simulink model "DLCReferenceApplication"  (R2018a)
settings: Solver=ode23tb  StartTime=0.0  StopTime=20  FixedStep=.001  RelTol=5e-3  EnableMultiTasking=on
StartFcn:
  | %tic
StopFcn:
  | %toc
model workspace (MAT data in the model file):
  A_mu = 10
  B_reff = 8.386
  Cz = 7766.25
  DCT_Param : struct (value not decoded)
  D_reff = 0.25826
  Downshift_Speeds = [9.5625 12.9375 16.3125 19.6875 23.0625 26.4375 29.8125 33.1875 36.5625 39.9375 43.3125 46.6875 ... (28 elements, 4x7)]
  Pedal_Positions = [0.1 0.4 0.5 0.9]
  SUS : struct (value not decoded)
  Upshift_Speeds = [12.9375 16.3125 19.6875 33 26.4375 29.8125 33.1875 52.5 39.9375 43.3125 46.6875 77.25 ... (28 elements, 4x7)]
  VEH : struct (value not decoded)
  V_o = 16.7
  V_xlow = 1
  WH : struct (value not decoded)
  a = 1.4
  alpha_max = 1.5
  alpha_min = -1.5
  b = 1.8
  c_zo = 209651
  epsilon = 0.1
  h = 0.134
  path : struct (value not decoded)
  pio = 220000
  q_Fcx = 0
  q_Fz2 = 15.4
  q_Fzy = 0
  q_reo = 0.9974
  q_sx1 = -0.007764
  q_sx10 = 0.2824
  q_sx11 = 5.349
  q_sx12 = 0
  q_sx13 = 0
  q_sx14 = 0
  q_sx2 = 1.1915
  q_sx3 = 0.013948
  q_sx4 = 4.912
  q_sx5 = 1.02
  q_sx6 = 22.83
  q_sx7 = 0.7104
  q_sx8 = -0.023393
  q_sx9 = 0.6581
  q_sy1 = 0.00702
  q_sy2 = 0
  q_sy3 = 0.001515
  q_sy4 = 8.514e-05
  q_sy5 = 0
  q_sy6 = 0
  q_sy7 = 0.9008
  q_sy8 = -0.4089
  q_v1 = 0.0007742
  q_v2 = 0.04667
  r_Bx1 = 12.531
  r_Bx2 = 9.532
  r_Bx3 = 0
  r_By1 = 10.615
  r_By2 = 7.705
  r_By3 = 3.433e-06
  r_By4 = 0
  r_Cx1 = 1.019
  r_Cy1 = 1.0585
  r_Ex1 = -0.4487
  r_Ex2 = -0.4726
  r_Ey1 = 0.3132
  r_Ey2 = 7.63e-06
  r_Hx1 = 0.0002374
  r_Hy1 = 0.011646
  r_Hy2 = 7.63e-06
  r_Vy1 = 0.05654
  r_Vy2 = 7.63e-06
  r_Vy3 = 0
  r_Vy4 = 99.9
  r_Vy5 = 2
  r_Vy6 = 15.814
  r_o = 0.3135
  vehWidth = 2
  w = 1
symbols that are objects in the model workspace (value not decoded): VEH
libraries: neural x286, simulink x5, sim3dlib x2, autolibutils x1, vehdynlibscenariocommon x1, vehdynlibdriver x1, vehdynlibviscommon x1
(part 13 of 13)

== system DLCReferenceApplication/Predictive Driver/Model Prediction Net/Layer 4/Delays 1 ==
  "p{4}" : Inport  PortDimensions=9
      mask Display: e = 0.06;c1 = [120 230 180]/255;c2 = ([120 230 180]+0)/(256+128);c3 = ([120 230 180]+128)/(256+128);patch([0 1 1 0],[0 0 1 1],c1);patch([0 1 1 1-e 1-e 0+e],[0 0 1 1-e 0+e 0+e],c2);patch([0 0 1 1-e 0+e 0+e],[0 1 1 1-e 1-e 0+e],c3);plot([0 1 1 0 0],[0 0 1 1 0]);
  mux : Mux  Inputs=1
      mask Display: e = 0.06;c1 = [120 150 230]/255;c2 = ([120 150 230]+0)/383;c3 = ([120 150 230]+128)/383;patch([0 1 1 0],[0 0 1 1],c1);patch([0 1 1 1-e 1-e 0+e],[0 0 1 1-e 0+e 0+e],c2);patch([0 0 1 1-e 0+e 0+e],[0 1 1 1-e 1-e 0+e],c3);plot([0 1 1 0 0],[0 0 1 1 0]);disp('Mux')
  "pd{4,1}" : Outport
      mask Display: e = 0.06;c1 = [120 230 180]/255;c2 = ([120 230 180]+0)/(256+128);c3 = ([120 230 180]+128)/(256+128);patch([0 1 1 0],[0 0 1 1],c1);patch([0 1 1 1-e 1-e 0+e],[0 0 1 1-e 0+e 0+e],c2);patch([0 0 1 1-e 0+e 0+e],[0 1 1 1-e 1-e 0+e],c3);plot([0 1 1 0 0],[0 0 1 1 0]);
  wires:
  "p{4}"/1 -> mux/1
  mux/1 -> "pd{4,1}"/1

== system DLCReferenceApplication/Predictive Driver/Model Prediction Net/Layer 4/Delays 2 ==
  "p{4}" : Inport  PortDimensions=20
      mask Display: e = 0.06;c1 = [120 230 180]/255;c2 = ([120 230 180]+0)/(256+128);c3 = ([120 230 180]+128)/(256+128);patch([0 1 1 0],[0 0 1 1],c1);patch([0 1 1 1-e 1-e 0+e],[0 0 1 1-e 0+e 0+e],c2);patch([0 0 1 1-e 0+e 0+e],[0 1 1 1-e 1-e 0+e],c3);plot([0 1 1 0 0],[0 0 1 1 0]);
  mux : Mux  Inputs=1
      mask Display: e = 0.06;c1 = [120 150 230]/255;c2 = ([120 150 230]+0)/383;c3 = ([120 150 230]+128)/383;patch([0 1 1 0],[0 0 1 1],c1);patch([0 1 1 1-e 1-e 0+e],[0 0 1 1-e 0+e 0+e],c2);patch([0 0 1 1-e 0+e 0+e],[0 1 1 1-e 1-e 0+e],c3);plot([0 1 1 0 0],[0 0 1 1 0]);disp('Mux')
  "pd{4,1}" : Outport
      mask Display: e = 0.06;c1 = [120 230 180]/255;c2 = ([120 230 180]+0)/(256+128);c3 = ([120 230 180]+128)/(256+128);patch([0 1 1 0],[0 0 1 1],c1);patch([0 1 1 1-e 1-e 0+e],[0 0 1 1-e 0+e 0+e],c2);patch([0 0 1 1-e 0+e 0+e],[0 1 1 1-e 1-e 0+e],c3);plot([0 1 1 0 0],[0 0 1 1 0]);
  wires:
  "p{4}"/1 -> mux/1
  mux/1 -> "pd{4,1}"/1

== system DLCReferenceApplication/Predictive Driver/Model Prediction Net/Layer 4/Delays 3 ==
  "p{4}" : Inport  PortDimensions=40
      mask Display: e = 0.06;c1 = [120 230 180]/255;c2 = ([120 230 180]+0)/(256+128);c3 = ([120 230 180]+128)/(256+128);patch([0 1 1 0],[0 0 1 1],c1);patch([0 1 1 1-e 1-e 0+e],[0 0 1 1-e 0+e 0+e],c2);patch([0 0 1 1-e 0+e 0+e],[0 1 1 1-e 1-e 0+e],c3);plot([0 1 1 0 0],[0 0 1 1 0]);
  mux : Mux  Inputs=1
      mask Display: e = 0.06;c1 = [120 150 230]/255;c2 = ([120 150 230]+0)/383;c3 = ([120 150 230]+128)/383;patch([0 1 1 0],[0 0 1 1],c1);patch([0 1 1 1-e 1-e 0+e],[0 0 1 1-e 0+e 0+e],c2);patch([0 0 1 1-e 0+e 0+e],[0 1 1 1-e 1-e 0+e],c3);plot([0 1 1 0 0],[0 0 1 1 0]);disp('Mux')
  "pd{4,2}" : Outport
      mask Display: e = 0.06;c1 = [120 230 180]/255;c2 = ([120 230 180]+0)/(256+128);c3 = ([120 230 180]+128)/(256+128);patch([0 1 1 0],[0 0 1 1],c1);patch([0 1 1 1-e 1-e 0+e],[0 0 1 1-e 0+e 0+e],c2);patch([0 0 1 1-e 0+e 0+e],[0 1 1 1-e 1-e 0+e],c3);plot([0 1 1 0 0],[0 0 1 1 0]);
  wires:
  "p{4}"/1 -> mux/1
  mux/1 -> "pd{4,2}"/1

== system DLCReferenceApplication/Predictive Driver/Model Prediction Net/Layer 4/Delays 4 ==
  "p{4}" : Inport  PortDimensions=20
      mask Display: e = 0.06;c1 = [120 230 180]/255;c2 = ([120 230 180]+0)/(256+128);c3 = ([120 230 180]+128)/(256+128);patch([0 1 1 0],[0 0 1 1],c1);patch([0 1 1 1-e 1-e 0+e],[0 0 1 1-e 0+e 0+e],c2);patch([0 0 1 1-e 0+e 0+e],[0 1 1 1-e 1-e 0+e],c3);plot([0 1 1 0 0],[0 0 1 1 0]);
  mux : Mux  Inputs=1
      mask Display: e = 0.06;c1 = [120 150 230]/255;c2 = ([120 150 230]+0)/383;c3 = ([120 150 230]+128)/383;patch([0 1 1 0],[0 0 1 1],c1);patch([0 1 1 1-e 1-e 0+e],[0 0 1 1-e 0+e 0+e],c2);patch([0 0 1 1-e 0+e 0+e],[0 1 1 1-e 1-e 0+e],c3);plot([0 1 1 0 0],[0 0 1 1 0]);disp('Mux')
  "pd{4,3}" : Outport
      mask Display: e = 0.06;c1 = [120 230 180]/255;c2 = ([120 230 180]+0)/(256+128);c3 = ([120 230 180]+128)/(256+128);patch([0 1 1 0],[0 0 1 1],c1);patch([0 1 1 1-e 1-e 0+e],[0 0 1 1-e 0+e 0+e],c2);patch([0 0 1 1-e 0+e 0+e],[0 1 1 1-e 1-e 0+e],c3);plot([0 1 1 0 0],[0 0 1 1 0]);
  wires:
  "p{4}"/1 -> mux/1
  mux/1 -> "pd{4,3}"/1

== system DLCReferenceApplication/Predictive Driver/Model Prediction Net/Layer 4/IW{4,1} ==
  "pd{4,1}" : Inport  PortDimensions=9
      mask Display: e = 0.06;c1 = [120 230 180]/255;c2 = ([120 230 180]+0)/(256+128);c3 = ([120 230 180]+128)/(256+128);patch([0 1 1 0],[0 0 1 1],c1);patch([0 1 1 1-e 1-e 0+e],[0 0 1 1-e 0+e 0+e],c2);patch([0 0 1 1-e 0+e 0+e],[0 1 1 1-e 1-e 0+e],c3);plot([0 1 1 0 0],[0 0 1 1 0]);
  "IW{4,1}(1,:)'" : Constant  Value=[-0.5771230834189629010921862573013640940189361572265625;-0.61619201660164957257137530177715234458446502685546875;-0.3922129123495980973501673361170105636119842529296875;0.475137795096655823900988480090745724737644195556640625;0.207635780743493703059954214040772058069705963134765625;-0.391896217881100461521981515033985488116741180419921875;0.9160420222304281878678011707961559295654296875;0.2452005034204982891754553975260932929813861846923828125;-0.4981323816541636251287172854063101112842559814453125]
      mask Display: e = 0.06;c1 = [120 150 230]/255;c2 = ([120 150 230]+0)/383;c3 = ([120 150 230]+128)/383;patch([0 1 1 0],[0 0 1 1],c1);patch([0 1 1 1-e 1-e 0+e],[0 0 1 1-e 0+e 0+e],c2);patch([0 0 1 1-e 0+e 0+e],[0 1 1 1-e 1-e 0+e],c3);plot([0 1 1 0 0],[0 0 1 1 0]);disp('Weights');
  Mux : Mux  Inputs=1
      mask Display: e = 0.06;c1 = [120 150 230]/255;c2 = ([120 150 230]+0)/383;c3 = ([120 150 230]+128)/383;patch([0 1 1 0],[0 0 1 1],c1);patch([0 1 1 1-e 1-e 0+e],[0 0 1 1-e 0+e 0+e],c2);patch([0 0 1 1-e 0+e 0+e],[0 1 1 1-e 1-e 0+e],c3);plot([0 1 1 0 0],[0 0 1 1 0]);disp('Mux');
  dotprod1 : neural/Weight Functions/dotprod
  "iz{4,1}" : Outport
      mask Display: e = 0.06;c1 = [120 230 180]/255;c2 = ([120 230 180]+0)/(256+128);c3 = ([120 230 180]+128)/(256+128);patch([0 1 1 0],[0 0 1 1],c1);patch([0 1 1 1-e 1-e 0+e],[0 0 1 1-e 0+e 0+e],c2);patch([0 0 1 1-e 0+e 0+e],[0 1 1 1-e 1-e 0+e],c3);plot([0 1 1 0 0],[0 0 1 1 0]);
  wires:
  "IW{4,1}(1,:)'"/1 -> dotprod1/1
  "pd{4,1}"/1 -> dotprod1/2
  dotprod1/1 -> Mux/1
  Mux/1 -> "iz{4,1}"/1

== system DLCReferenceApplication/Predictive Driver/Model Prediction Net/Layer 4/LW{4,1} ==
  "ad{4,1}" : Inport  PortDimensions=20
      mask Display: e = 0.06;c1 = [120 230 180]/255;c2 = ([120 230 180]+0)/(256+128);c3 = ([120 230 180]+128)/(256+128);patch([0 1 1 0],[0 0 1 1],c1);patch([0 1 1 1-e 1-e 0+e],[0 0 1 1-e 0+e 0+e],c2);patch([0 0 1 1-e 0+e 0+e],[0 1 1 1-e 1-e 0+e],c3);plot([0 1 1 0 0],[0 0 1 1 0]);
  "IW{4,1}(1,:)'" : Constant  Value=[0.916684685790865483312472861143760383129119873046875;0.2636851771929895615897976313135586678981781005859375;-0.3492331089734814764113934870692901313304901123046875;-0.11786503709245825521900741250647115521132946014404296875;0.50320078446947380523823767362046055495738983154296875;-0.4927000401571077770057627276401035487651824951171875;-0.2088832457984179657994872059134650044143199920654296875;0.4465785632290864004545483112451620399951934814453125;0.10461125196919902891057319038736750371754169464111328125;-0.0427743850947984449728522804434760473668575286865234375;0.405797206791189746244441494127386249601840972900390625;-0.43662126395722722360659417972783558070659637451171875;-0.181658127076019193513189975419663824141025543212890625;0.41899883394469272790416880525299347937107086181640625;-0.533044452130733592554179267608560621738433837890625;0.16098318242033993197281915854546241462230682373046875;-0.219792476259432822960349085406051017343997955322265625;-0.426441538733121794368940982167259790003299713134765625;0.09693073801308534076515144306540605612099170684814453125;-0.0290423415959079438131151817970021511428058147430419921875]
      mask Display: e = 0.06;c1 = [120 150 230]/255;c2 = ([120 150 230]+0)/383;c3 = ([120 150 230]+128)/383;patch([0 1 1 0],[0 0 1 1],c1);patch([0 1 1 1-e 1-e 0+e],[0 0 1 1-e 0+e 0+e],c2);patch([0 0 1 1-e 0+e 0+e],[0 1 1 1-e 1-e 0+e],c3);plot([0 1 1 0 0],[0 0 1 1 0]);disp('weights');
  Mux : Mux  Inputs=1
      mask Display: e = 0.06;c1 = [120 150 230]/255;c2 = ([120 150 230]+0)/383;c3 = ([120 150 230]+128)/383;patch([0 1 1 0],[0 0 1 1],c1);patch([0 1 1 1-e 1-e 0+e],[0 0 1 1-e 0+e 0+e],c2);patch([0 0 1 1-e 0+e 0+e],[0 1 1 1-e 1-e 0+e],c3);plot([0 1 1 0 0],[0 0 1 1 0]);disp('Mux');
  dotprod1 : neural/Weight Functions/dotprod
  "lz{4,1}" : Outport
      mask Display: e = 0.06;c1 = [120 230 180]/255;c2 = ([120 230 180]+0)/(256+128);c3 = ([120 230 180]+128)/(256+128);patch([0 1 1 0],[0 0 1 1],c1);patch([0 1 1 1-e 1-e 0+e],[0 0 1 1-e 0+e 0+e],c2);patch([0 0 1 1-e 0+e 0+e],[0 1 1 1-e 1-e 0+e],c3);plot([0 1 1 0 0],[0 0 1 1 0]);
  wires:
  "IW{4,1}(1,:)'"/1 -> dotprod1/1
  "ad{4,1}"/1 -> dotprod1/2
  dotprod1/1 -> Mux/1
  Mux/1 -> "lz{4,1}"/1

== system DLCReferenceApplication/Predictive Driver/Model Prediction Net/Layer 4/LW{4,2} ==
  "ad{4,2}" : Inport  PortDimensions=40
      mask Display: e = 0.06;c1 = [120 230 180]/255;c2 = ([120 230 180]+0)/(256+128);c3 = ([120 230 180]+128)/(256+128);patch([0 1 1 0],[0 0 1 1],c1);patch([0 1 1 1-e 1-e 0+e],[0 0 1 1-e 0+e 0+e],c2);patch([0 0 1 1-e 0+e 0+e],[0 1 1 1-e 1-e 0+e],c3);plot([0 1 1 0 0],[0 0 1 1 0]);
  "IW{4,2}(1,:)'" : Constant  Value=[0.27949113896556332381493348293588496744632720947265625;-0.64821034904210217408859762144857086241245269775390625;-0.31207165074660492276592549387714825570583343505859375;0.68179045523777859205694085176219232380390167236328125;0.1070962845116746053886203071670024655759334564208984375;0.71796848345370090083150671489420346915721893310546875;0.41775067515994901423681540109100751578807830810546875;-0.07416614077972365215440930796830798499286174774169921875;-0.317614313441147821936993977942620404064655303955078125;0.17180598844553951476399333841982297599315643310546875;0.61751675691226182163262592439423315227031707763671875;0.7716454001251751293466440984047949314117431640625;0.628633241433649292417840115376748144626617431640625;-0.476268167532110597850447675227769650518894195556640625;-0.6502480025402694874259168500429950654506683349609375;0.30243377430933848781791084547876380383968353271484375;0.844839423767121733277463135891593992710113525390625;0.373547457832598350790931363007985055446624755859375;-0.80117493041453047286637456636526621878147125244140625;0.60554222667279322678268727031536400318145751953125;0.059121620432629869157370450238886405713856220245361328125;0.497651004579527767024416107233264483511447906494140625;-0.054601145604125940480333412097024847753345966339111328125;0.329012943235255816976092546610743738710880279541015625;-0.664841453781237046172236659913323819637298583984375;-0.930814332006292932675250995089299976825714111328125;0.75058269710626868143066303673549555242061614990234375;0.374191155045953627311661193743930198252201080322265625;-0.269357044111559196242211555727408267557621002197265625;0.55546512678121839901024259233963675796985626220703125;-0.82428439513931228699306075213826261460781097412109375;0.11409778951636805055525059060528292320668697357177734375;-0.20589850521900998625568490751902572810649871826171875;-0.96061551361853603214768781981547363102436065673828125;-0.6617327123586644876951368132722564041614532470703125;-0.57015635361925609547739668414578773081302642822265625;0.1170755103561895993369290636110235936939716339111328125;-0.97609141183504932737236003958969376981258392333984375;0.372523900286641673762488835563999600708484649658203125;0.0921821536508019845346240117578417994081974029541015625]
      mask Display: e = 0.06;c1 = [120 150 230]/255;c2 = ([120 150 230]+0)/383;c3 = ([120 150 230]+128)/383;patch([0 1 1 0],[0 0 1 1],c1);patch([0 1 1 1-e 1-e 0+e],[0 0 1 1-e 0+e 0+e],c2);patch([0 0 1 1-e 0+e 0+e],[0 1 1 1-e 1-e 0+e],c3);plot([0 1 1 0 0],[0 0 1 1 0]);disp('weights');
  Mux : Mux  Inputs=1
      mask Display: e = 0.06;c1 = [120 150 230]/255;c2 = ([120 150 230]+0)/383;c3 = ([120 150 230]+128)/383;patch([0 1 1 0],[0 0 1 1],c1);patch([0 1 1 1-e 1-e 0+e],[0 0 1 1-e 0+e 0+e],c2);patch([0 0 1 1-e 0+e 0+e],[0 1 1 1-e 1-e 0+e],c3);plot([0 1 1 0 0],[0 0 1 1 0]);disp('Mux');
  dotprod1 : neural/Weight Functions/dotprod
  "lz{4,2}" : Outport
      mask Display: e = 0.06;c1 = [120 230 180]/255;c2 = ([120 230 180]+0)/(256+128);c3 = ([120 230 180]+128)/(256+128);patch([0 1 1 0],[0 0 1 1],c1);patch([0 1 1 1-e 1-e 0+e],[0 0 1 1-e 0+e 0+e],c2);patch([0 0 1 1-e 0+e 0+e],[0 1 1 1-e 1-e 0+e],c3);plot([0 1 1 0 0],[0 0 1 1 0]);
  wires:
  "IW{4,2}(1,:)'"/1 -> dotprod1/1
  "ad{4,2}"/1 -> dotprod1/2
  dotprod1/1 -> Mux/1
  Mux/1 -> "lz{4,2}"/1

== system DLCReferenceApplication/Predictive Driver/Model Prediction Net/Layer 4/LW{4,3} ==
  "ad{4,3}" : Inport  PortDimensions=20
      mask Display: e = 0.06;c1 = [120 230 180]/255;c2 = ([120 230 180]+0)/(256+128);c3 = ([120 230 180]+128)/(256+128);patch([0 1 1 0],[0 0 1 1],c1);patch([0 1 1 1-e 1-e 0+e],[0 0 1 1-e 0+e 0+e],c2);patch([0 0 1 1-e 0+e 0+e],[0 1 1 1-e 1-e 0+e],c3);plot([0 1 1 0 0],[0 0 1 1 0]);
  "IW{4,3}(1,:)'" : Constant  Value=[-0.1628349878900283709270979670691303908824920654296875;0.81751526230570359388138967915438115596771240234375;-0.496913605383706047380343306940631009638309478759765625;-0.2429698308711668863768551318571553565561771392822265625;-0.326261663138057877997511013745679520070552825927734375;-0.51423468523078452729890841510496102273464202880859375;0.93183964004850994289341770127066411077976226806640625;1.06220128464347052243965663365088403224945068359375;0.331727610839852637969471516043995507061481475830078125;-0.6576225313520505100228774608694948256015777587890625;0.363097376670315996616267284480272792279720306396484375;0.65638555479970606132411603539367206394672393798828125;0.60023274740255361248131293905316852033138275146484375;-1.0283452056308408639750950896996073424816131591796875;0.1790768619482399903741765001541352830827236175537109375;-0.57978484994542245356541343426215462386608123779296875;0.77240696146937304344959329682751558721065521240234375;-0.49470338241571620851999568913015536963939666748046875;0.81095602974825087283505808954942040145397186279296875;1.03775966828370602712539039202965795993804931640625]
      mask Display: e = 0.06;c1 = [120 150 230]/255;c2 = ([120 150 230]+0)/383;c3 = ([120 150 230]+128)/383;patch([0 1 1 0],[0 0 1 1],c1);patch([0 1 1 1-e 1-e 0+e],[0 0 1 1-e 0+e 0+e],c2);patch([0 0 1 1-e 0+e 0+e],[0 1 1 1-e 1-e 0+e],c3);plot([0 1 1 0 0],[0 0 1 1 0]);disp('weights');
  Mux : Mux  Inputs=1
      mask Display: e = 0.06;c1 = [120 150 230]/255;c2 = ([120 150 230]+0)/383;c3 = ([120 150 230]+128)/383;patch([0 1 1 0],[0 0 1 1],c1);patch([0 1 1 1-e 1-e 0+e],[0 0 1 1-e 0+e 0+e],c2);patch([0 0 1 1-e 0+e 0+e],[0 1 1 1-e 1-e 0+e],c3);plot([0 1 1 0 0],[0 0 1 1 0]);disp('Mux');
  dotprod1 : neural/Weight Functions/dotprod
  "lz{4,3}" : Outport
      mask Display: e = 0.06;c1 = [120 230 180]/255;c2 = ([120 230 180]+0)/(256+128);c3 = ([120 230 180]+128)/(256+128);patch([0 1 1 0],[0 0 1 1],c1);patch([0 1 1 1-e 1-e 0+e],[0 0 1 1-e 0+e 0+e],c2);patch([0 0 1 1-e 0+e 0+e],[0 1 1 1-e 1-e 0+e],c3);plot([0 1 1 0 0],[0 0 1 1 0]);
  wires:
  "IW{4,3}(1,:)'"/1 -> dotprod1/1
  "ad{4,3}"/1 -> dotprod1/2
  dotprod1/1 -> Mux/1
  Mux/1 -> "lz{4,3}"/1

== system DLCReferenceApplication/Visualization/3D Engine/3D Engine/Part Rotation Concatenation ==
  Body Roll : Inport
  Body Ptich : Inport  Port=2
  Body Yaw : Inport  Port=3
  WheelFrontLeft Pitch : Inport  Port=4
  WheelFrontRight Pitch : Inport  Port=5
  WheelRearLeft Pitch : Inport  Port=6
  WheelRearRight Ptich : Inport  Port=7
  WheelFrontLeft Roll : Inport  Port=8
  WheelFrontRight Roll : Inport  Port=9
  WheelRearLeft Roll : Inport  Port=10
  WheelRearRight Roll : Inport  Port=11
  WheelFrontLeft Yaw : Inport  Port=12
  WheelFrontRight Yaw : Inport  Port=13
  WheelRearLeft Yaw : Inport  Port=14
  WheelRearRight Yaw : Inport  Port=15
  AllParts : Concatenate  NumInputs=5  Mode=Multidimensional array
  Body : Concatenate  NumInputs=3  Mode=Multidimensional array  ConcatenateDimension=2
  WheelFrontLeft : Concatenate  NumInputs=3  Mode=Multidimensional array  ConcatenateDimension=2
  WheelFrontRight : Concatenate  NumInputs=3  Mode=Multidimensional array  ConcatenateDimension=2
  WheelRearLeft : Concatenate  NumInputs=3  Mode=Multidimensional array  ConcatenateDimension=2
  WheelRearRight : Concatenate  NumInputs=3  Mode=Multidimensional array  ConcatenateDimension=2
  ConcatOut : Outport
  wires:
  WheelFrontRight Yaw/1 -> WheelFrontRight/3
  WheelRearLeft Pitch/1 -> WheelRearLeft/1
  WheelRearRight/1 -> AllParts/5
  WheelRearLeft Roll/1 -> WheelRearLeft/2
  AllParts/1 -> ConcatOut/1
  WheelRearLeft Yaw/1 -> WheelRearLeft/3
  WheelRearRight Roll/1 -> WheelRearRight/2
  WheelFrontRight Pitch/1 -> WheelFrontRight/1
  WheelFrontRight Roll/1 -> WheelFrontRight/2
  WheelRearRight Yaw/1 -> WheelRearRight/3
  WheelFrontRight/1 -> AllParts/3
  WheelRearLeft/1 -> AllParts/4
  Body/1 -> AllParts/1
  WheelRearRight Ptich/1 -> WheelRearRight/1
  WheelFrontLeft/1 -> AllParts/2
  Body Roll/1 -> Body/2
  WheelFrontLeft Roll/1 -> WheelFrontLeft/2
  WheelFrontLeft Yaw/1 -> WheelFrontLeft/3
  WheelFrontLeft Pitch/1 -> WheelFrontLeft/1
  Body Yaw/1 -> Body/3
  Body Ptich/1 -> Body/1

== system DLCReferenceApplication/Visualization/3D Engine/3D Engine/Part Translation Concatenation ==
  BodyX : Inport
  BodyY : Inport  Port=2
  BodyZ : Inport  Port=3
  WheelFrontLeftX : Inport  Port=4
  WheelFrontRightX : Inport  Port=5
  WheelRearLeftX : Inport  Port=6
  WheelRearRightX : Inport  Port=7
  WheelFrontLeftY : Inport  Port=8
  WheelFrontRightY : Inport  Port=9
  WheelRearLeftY : Inport  Port=10
  WheelRearRightY : Inport  Port=11
  WheelFrontLeftZ : Inport  Port=12
  WheelFrontRightZ : Inport  Port=13
  WheelRearLeftZ : Inport  Port=14
  WheelRearRightZ : Inport  Port=15
  AllParts : Concatenate  NumInputs=5  Mode=Multidimensional array
  Body : Concatenate  NumInputs=3  Mode=Multidimensional array  ConcatenateDimension=2
  WheelFrontLeft : Concatenate  NumInputs=3  Mode=Multidimensional array  ConcatenateDimension=2
  WheelFrontRight : Concatenate  NumInputs=3  Mode=Multidimensional array  ConcatenateDimension=2
  WheelRearLeft : Concatenate  NumInputs=3  Mode=Multidimensional array  ConcatenateDimension=2
  WheelRearRight : Concatenate  NumInputs=3  Mode=Multidimensional array  ConcatenateDimension=2
  ConcatOut : Outport
  wires:
  WheelFrontRightZ/1 -> WheelFrontRight/3
  WheelRearLeftX/1 -> WheelRearLeft/1
  WheelRearRight/1 -> AllParts/5
  WheelRearLeftY/1 -> WheelRearLeft/2
  AllParts/1 -> ConcatOut/1
  WheelRearLeftZ/1 -> WheelRearLeft/3
  WheelRearRightY/1 -> WheelRearRight/2
  WheelFrontRightX/1 -> WheelFrontRight/1
  WheelFrontRightY/1 -> WheelFrontRight/2
  WheelRearRightZ/1 -> WheelRearRight/3
  WheelFrontRight/1 -> AllParts/3
  WheelRearLeft/1 -> AllParts/4
  Body/1 -> AllParts/1
  WheelRearRightX/1 -> WheelRearRight/1
  WheelFrontLeft/1 -> AllParts/2
  BodyY/1 -> Body/2
  WheelFrontLeftY/1 -> WheelFrontLeft/2
  WheelFrontLeftZ/1 -> WheelFrontLeft/3
  WheelFrontLeftX/1 -> WheelFrontLeft/1
  BodyZ/1 -> Body/3
  BodyX/1 -> Body/1

== system DLCReferenceApplication/Visualization/3D Engine/3D Engine/Scale ==
  Constant{1..12,17,32..33} (15 alike) : Constant  OutDataTypeStr=single
  PartConcatenation : Subsystem
  ScaleOut : Outport
  wires:
  PartConcatenation/1(ConcatOut) -> ScaleOut/1
  Constant12/1 -> PartConcatenation/1(BodyX)
  Constant17/1 -> PartConcatenation/2(BodyY)
  Constant32/1 -> PartConcatenation/3(BodyZ)
  Constant33/1 -> PartConcatenation/4(WheelFrontLeftX)
  Constant1/1 -> PartConcatenation/5(WheelFrontLeftY)
  Constant2/1 -> PartConcatenation/6(WheelFrontLeftZ)
  Constant5/1 -> PartConcatenation/7(WheelFrontRightX)
  Constant3/1 -> PartConcatenation/8(WheelFrontRightY)
  Constant4/1 -> PartConcatenation/9(WheelFrontRightZ)
  Constant8/1 -> PartConcatenation/10(WheelRearLeftX)
  Constant6/1 -> PartConcatenation/11(WheelRearLeftY)
  Constant7/1 -> PartConcatenation/12(WheelRearLeftZ)
  Constant11/1 -> PartConcatenation/13(WheelRearRightX)
  Constant9/1 -> PartConcatenation/14(WheelRearRightY)
  Constant10/1 -> PartConcatenation/15(WheelRearRightZ)

== system DLCReferenceApplication/Controllers/Brake Controller/Brake Pressure Control/Bang Bang ABS/Bang-bang controller ==
  in_1 : Inport
  Constant : Constant  Value=0
  Data Type Conversion1 : DataTypeConversion  OutDataTypeStr=double  SaturateOnIntegerOverflow=on  RndMeth=Zero
  Data Type Conversion2 : DataTypeConversion  OutDataTypeStr=double  SaturateOnIntegerOverflow=on  RndMeth=Zero
  Relational Operator : RelationalOperator  Operator=>  OutDataTypeStr=boolean  RndMeth=Nearest  InputSameDT=on
  Relational Operator1 : RelationalOperator  Operator=<  OutDataTypeStr=boolean  RndMeth=Nearest  InputSameDT=on
  Sum : Sum  Inputs=+-  SaturateOnIntegerOverflow=on  InputSameDT=on  OutDataTypeStr=Inherit: Same as first input
  out_1 : Outport  InitialOutput=0
  wires:
  Data Type Conversion2/1 -> Sum/2
  Data Type Conversion1/1 -> Sum/1
  Sum/1 -> out_1/1
  Relational Operator/1 -> Data Type Conversion1/1
  Relational Operator1/1 -> Data Type Conversion2/1
  Constant/1 -> Relational Operator/2, Relational Operator1/2
  in_1/1 -> Relational Operator1/1, Relational Operator/1

== system DLCReferenceApplication/Visualization/3D Engine/3D Engine/Scale/PartConcatenation ==
  BodyX : Inport
  BodyY : Inport  Port=2
  BodyZ : Inport  Port=3
  WheelFrontLeftX : Inport  Port=4
  WheelFrontLeftY : Inport  Port=5
  WheelFrontLeftZ : Inport  Port=6
  WheelFrontRightX : Inport  Port=7
  WheelFrontRightY : Inport  Port=8
  WheelFrontRightZ : Inport  Port=9
  WheelRearLeftX : Inport  Port=10
  WheelRearLeftY : Inport  Port=11
  WheelRearLeftZ : Inport  Port=12
  WheelRearRightX : Inport  Port=13
  WheelRearRightY : Inport  Port=14
  WheelRearRightZ : Inport  Port=15
  AllParts : Concatenate  NumInputs=5  Mode=Multidimensional array
  Body : Concatenate  NumInputs=3  Mode=Multidimensional array  ConcatenateDimension=2
  WheelFrontLeft : Concatenate  NumInputs=3  Mode=Multidimensional array  ConcatenateDimension=2
  WheelFrontRight : Concatenate  NumInputs=3  Mode=Multidimensional array  ConcatenateDimension=2
  WheelRearLeft : Concatenate  NumInputs=3  Mode=Multidimensional array  ConcatenateDimension=2
  WheelRearRight : Concatenate  NumInputs=3  Mode=Multidimensional array  ConcatenateDimension=2
  ConcatOut : Outport
  wires:
  WheelFrontRightZ/1 -> WheelFrontRight/3
  WheelRearLeftX/1 -> WheelRearLeft/1
  WheelRearRight/1 -> AllParts/5
  WheelRearLeftY/1 -> WheelRearLeft/2
  AllParts/1 -> ConcatOut/1
  WheelRearLeftZ/1 -> WheelRearLeft/3
  WheelRearRightY/1 -> WheelRearRight/2
  WheelFrontRightX/1 -> WheelFrontRight/1
  WheelFrontRightY/1 -> WheelFrontRight/2
  WheelRearRightZ/1 -> WheelRearRight/3
  WheelFrontRight/1 -> AllParts/3
  WheelRearLeft/1 -> AllParts/4
  Body/1 -> AllParts/1
  WheelRearRightX/1 -> WheelRearRight/1
  WheelFrontLeft/1 -> AllParts/2
  BodyY/1 -> Body/2
  WheelFrontLeftY/1 -> WheelFrontLeft/2
  WheelFrontLeftZ/1 -> WheelFrontLeft/3
  WheelFrontLeftX/1 -> WheelFrontLeft/1
  BodyZ/1 -> Body/3
  BodyX/1 -> Body/1

== stateflow chart DLCReferenceApplication/Controllers/Transmission Controller/TCM/TCM Shift Controller ==
  settings: sampleTime=0.01
  state GearState [parallel]
    settings: executionOrder=1
    state Neutral
      en:
      GearState = 0;
    state G1
      en:
      GearState = 1;
    state G2
      en:
      GearState = 2;
      du:
      [SpdThr] = calc(2,pedal,speed);
    state G3
      en:
      GearState = 3;
      du:
      [SpdThr] = calc(3,pedal,speed);
    state G8
      en:
      GearState = 8;
    state G7
      en:
      GearState = 7;
    state G6
      en:
      GearState = 6;
    state G5
      en:GearState=5;
      du:[SpdThr]=calc(5,pedal,speed);
    state G4
      en:
      GearState = 4;
      du:
      [SpdThr] = calc(4,pedal,speed);
    (default) -> G1
    Neutral -> G1 : [~Neutral]
    G1 -> G2 [order 1] : Up
    G2 -> G3 [order 1] : Up
    G1 -> Neutral [order 2] : [Neutral]
    G2 -> G1 [order 2] : Down
    G3 -> G2 [order 2] : Down
    G3 -> G4 [order 1] : Up
    G4 -> G3 [order 2] : Down
    G7 -> G8 [order 1] : Up
    G5 -> G6 [order 1] : Up
    G6 -> G7 [order 1] : Up
    G4 -> G5 [order 1] : Up
    G5 -> G4 [order 2] : Down
    G6 -> G5 [order 2] : Down
    G7 -> G6 [order 2] : Down
    G8 -> G7 : Down
  state SelectionState [parallel]
    du:[up_th]=calc_up(GearState,pedal);
    du:[down_th]=calc_down(GearState,pedal);
    settings: executionOrder=2
    state SteadyState
      en:
      clutchControl = 0;
    state preDownShifting
    state preUpShifting
    state UpShifting
      en:
      GearState = GearState + 0.5;
    state DownShifting
      en:
      GearState = GearState - 0.5;
    (default) -> SteadyState
    SteadyState -> (junction 62) [order 1] : [speed < down_th && ...
        | GearState >1]
    SteadyState -> (junction 128) [order 2] : [speed > up_th &&...
        | GearState <= 5 && ...
        | floor(GearState) == GearState]
    (junction 62) -> preDownShifting
    (junction 128) -> preUpShifting
    (junction 168) -> SteadyState
    (junction 23) -> SteadyState
    (junction 161) -> SteadyState
    preDownShifting -> (junction 168) [order 2] : [speed >= down_th]
    preUpShifting -> (junction 161) [order 2] : [speed <= up_th]
    preUpShifting -> UpShifting [order 1] : after(0.5,sec)
        | [speed>up_th]
    preDownShifting -> DownShifting [order 1] : after(0.5, sec)
        | [speed < down_th - 2]
    DownShifting -> (junction 23) : {GearState.Down;}
    UpShifting -> (junction 23) : {GearState.Up;}
  state up_th = calc_up(gear,pedal) [function]
  state down_th = calc_down(gear,pedal) [function]
  state SpdThr = calc(gear,pedal,speed) [function]
  data: gear function_input; pedal function_input; up_th function_output; gear function_input; pedal function_input; down_th function_output; gear function_input; pedal function_input; SpdThr function_output; speed function_input; GearState output int8; speed input; pedal input; clutchControl local double; SpdThr local double; Neutral input; up_th local double; down_th local double
  events: Up local EITHER_EDGE_EVENT; Down local EITHER_EDGE_EVENT
